simulink model "BaitapBangBang"  (R2022a)
settings: Solver=FixedStepAuto  StartTime=0.0  StopTime=60  FixedStep=0.01  RelTol=1e-3  EnableMultiTasking=on
libraries: arduinolib x3, arduinosensorlib x1
settings Model: ExtModeTrigDuration=2  Creator=phong  LastModifiedBy=kietn
settings OptimizationCC: EnhancedBackFolding=on  PassReuseOutputArgsAs=Individual arguments  ZeroExternalMemoryAtStartup=off  ZeroInternalMemoryAtStartup=off  MaxStackSize=64  OptimizeBlockOrder=speed  DifferentSizesBufferReuse=on  OptimizationCustomize=off  EfficientTunableParamExpr=on
settings DebuggingCC: ParameterTunabilityLossMsg=error
settings HardwareCC: ProdBitPerPointer=32  ProdBitPerSizeT=32  ProdBitPerPtrDiffT=32  ProdLargestAtomicInteger=Long  ProdLargestAtomicFloat=Double  ProdWordSize=32  ProdHWDeviceType=ARM Compatible->ARM Cortex
settings SFSimCC: MATLABDynamicMemAlloc=off
settings RTWCC: SystemTargetFile=ert.tlc  HardwareBoard=ESP32-WROOM(Arduino Compatible)  TLCOptions="-aInlineSetEventsForThisBaseRateFcn=TLC_FALSE -aSuppressMultiTaskScheduler=TLC_FALSE  -aRateBasedStepFcn=0"  TemplateMakefile=ert_default_tmf  Toolchain=ESP32  BuildConfiguration=Faster Runs
settings CodeAppCC: ForceParamTrailComments=on  IgnoreCustomStorageClasses=off  OperatorAnnotations=on  SimulinkDataObjDesc=on  SFDataObjDesc=on  InsertBlockDesc=on
settings ERTTargetCC: SupportContinuousTime=on  SupportVariableSizeSignals=on  ExtModeTransport=3  ExtModeStaticAlloc=on  ExtModeStaticAllocSize=65536  ExtModeMexFile=ext_xcp  ExtModeIntrfLevel=Level2 - Open

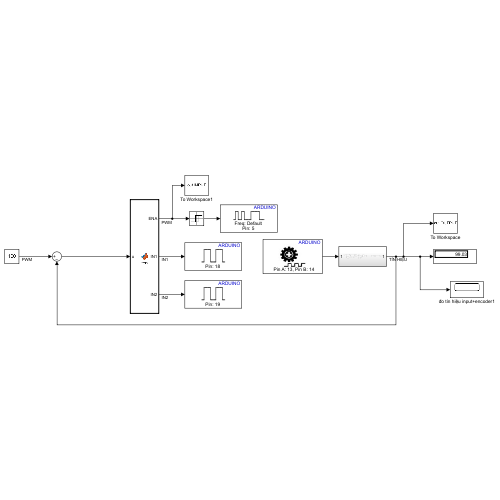
[thumbnail: Simulink's stored preview of the top-level diagram]
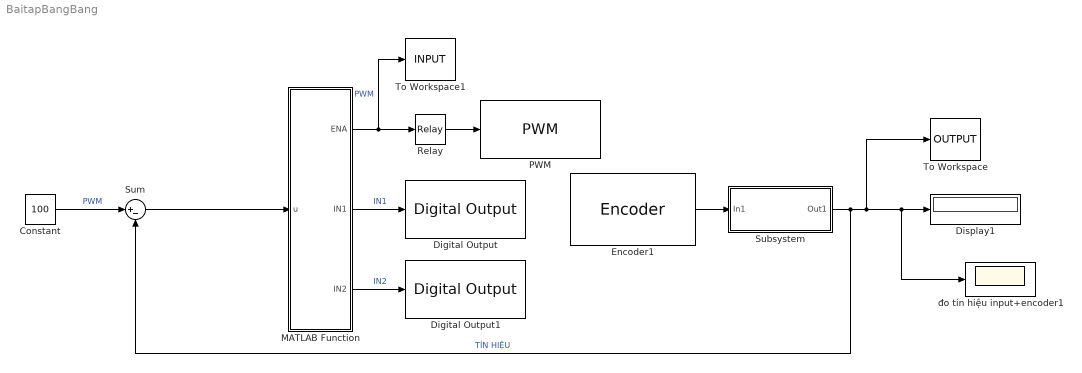
== system BaitapBangBang ==
  Constant : Constant  Value=100
  Digital Output : arduinolib/Digital Output  pinNumber=18  Direction=output  blockPlatform=arduino
  Digital Output1 : arduinolib/Digital Output  pinNumber=19  Direction=output  blockPlatform=arduino
  Display1 : Display
  Encoder1 : arduinosensorlib/Encoder  InputA=13  InputB=14  Mode=No reset  SampleTime=-1
      settings: SourceProductBaseCode=ARDUINO
  MATLAB Function : MATLAB Function  TreatAsAtomicUnit=on
  PWM : arduinolib/PWM  pinNumber=5  frequencyType=Default  desiredFrequency=490.2  achievableFrequency=490.2
  Relay : Relay  OnOutputValue=100
  Subsystem : Subsystem
  Sum : Sum  Inputs=|+-
  To Workspace : ToWorkspace  VariableName=OUTPUT  SampleTime=-1
      settings: Save2DSignal=2-D array (concatenate along first dimension)
  To Workspace1 : ToWorkspace  VariableName=INPUT  SampleTime=-1
      settings: Save2DSignal=2-D array (concatenate along first dimension)
  đo tín hiệu input+encoder1 : Scope
  wires:
  Encoder1/1 -> Subsystem/1(In1)
  Subsystem/1(Out1) -> Sum/2, To Workspace/1, đo tín hiệu input+encoder1/1, Display1/1  "TÍN HIỆU"
  MATLAB Function/1(ENA) -> To Workspace1/1, Relay/1  "PWM"
  MATLAB Function/2(IN1) -> Digital Output/1  "IN1"
  MATLAB Function/3(IN2) -> Digital Output1/1  "IN2"
  Constant/1 -> Sum/1  "PWM"
  Sum/1 -> MATLAB Function/1(u)
  Relay/1 -> PWM/1

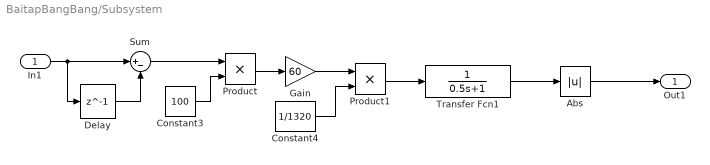
== system BaitapBangBang/Subsystem ==
  In1 : Inport
  Abs : Abs  SaturateOnIntegerOverflow=off
  Constant3 : Constant  Value=100
  Constant4 : Constant  Value=1/1320
  Delay : Delay  DelayLength=1
  Gain : Gain  Gain=60
  Product : Product
  Product1 : Product  OutDataTypeStr=double
  Sum : Sum  Inputs=|+-
  Transfer Fcn1 : TransferFcn  Denominator=[0.5 1]
  Out1 : Outport
  wires:
  Constant4/1 -> Product1/2
  In1/1 -> Sum/1, Delay/1
  Constant3/1 -> Product/2
  Sum/1 -> Product/1
  Delay/1 -> Sum/2
  Gain/1 -> Product1/1
  Product/1 -> Gain/1
  Product1/1 -> Transfer Fcn1/1
  Transfer Fcn1/1 -> Abs/1
  Abs/1 -> Out1/1

== matlab function BaitapBangBang/MATLAB Function ==
  data: u input; ENA output; IN1 output; IN2 output
function [ENA,IN1,IN2] = fcn(u)

ENA=abs(u);
if u<0 
    IN1=1; IN2=0;
elseif u>0
    IN1=0; IN2=1;
else 
    IN1=0; IN2=0;
end
